simulink model "localMapServer"  (R2024a)
settings: Solver=FixedStepAuto  StartTime=0.0  StopTime=inf  RelTol=1e-3
model workspace (MAT data in the model file):
  SL_ROS_VariableLengthArrays_MaxSizes.CommonInfo.ArrayTruncateAction = 'EmitWarning'
  SL_ROS_VariableLengthArrays_MaxSizes.MsgTypeMap = containers.Map
  SL_ROS_VariableLengthArrays_MaxSizes.MsgTypeMap.serialization.keys = {'std_msgs/Int8MultiArray'}
  SL_ROS_VariableLengthArrays_MaxSizes.MsgTypeMap.serialization.values{1}.PropertyName = 'data'
  SL_ROS_VariableLengthArrays_MaxSizes.MsgTypeMap.serialization.values{1}.DataType = 'int8'
  SL_ROS_VariableLengthArrays_MaxSizes.MsgTypeMap.serialization.values{1}.MaxLength = 1500000
  SL_ROS_VariableLengthArrays_MaxSizes.MsgTypeMap.serialization.uniformity = 0
  SL_ROS_VariableLengthArrays_MaxSizes.MsgTypeMap.serialization.keyType = 'char'
  SL_ROS_VariableLengthArrays_MaxSizes.MsgTypeMap.serialization.valueType = 'any'
undefined symbols (not defined in the file): egogridsize, egomat, egores, gridloc
libraries: roshelperlib x2, ros2lib x2, simulink x1
settings Model: Creator=cstabile  LastModifiedBy=cstabile
settings OptimizationCC: EnhancedBackFolding=on  PassReuseOutputArgsAs=Individual arguments  ZeroExternalMemoryAtStartup=off  ZeroInternalMemoryAtStartup=off  MaxStackSize=64  OptimizeBlockOrder=speed  DifferentSizesBufferReuse=on  OptimizationCustomize=off  EfficientTunableParamExpr=on
settings DebuggingCC: ParameterTunabilityLossMsg=error
settings SFSimCC: MATLABDynamicMemAlloc=off
settings RTWCC: Description=Embedded Coder  SystemTargetFile=ert.tlc  HardwareBoard=Robot Operating System 2 (ROS 2)  TLCOptions="-aInlineSetEventsForThisBaseRateFcn=TLC_FALSE -aSuppressMultiTaskScheduler=TLC_FALSE  -aRateBasedStepFcn=0"  TemplateMakefile=ert_default_tmf  Toolchain=Colcon Tools  TargetLang=C++
settings CodeAppCC: ForceParamTrailComments=on  IgnoreCustomStorageClasses=off  OperatorAnnotations=on  SimulinkDataObjDesc=on  SFDataObjDesc=on  InsertBlockDesc=on
settings ERTTargetCC: CodeInterfacePackaging=C++ class  RootIOFormat=Structure reference

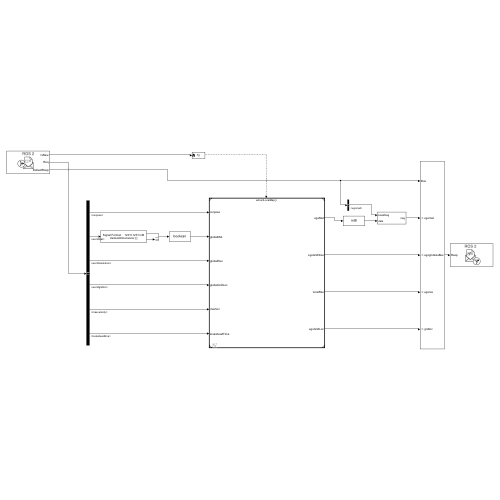
[thumbnail: Simulink's stored preview of the top-level diagram]
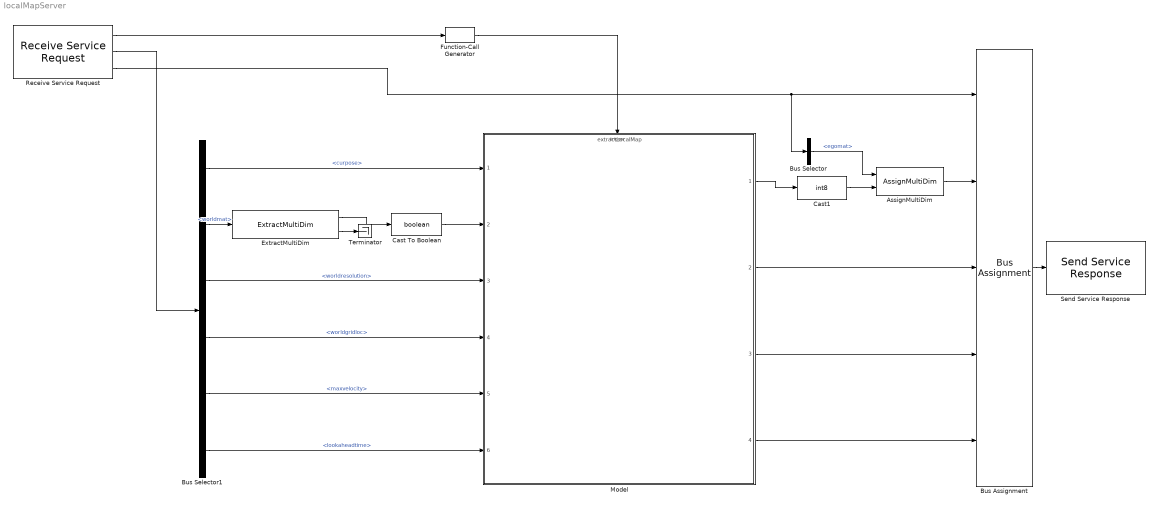
== system localMapServer ==
  AssignMultiDim : roshelperlib/AssignMultiDim  SystemSampleTime=-1  VariantActivationTime=update diagram  AllowFlexibleInterface=on  Latency=0  AutoFrameSizeCalculation=off
  Bus Assignment : BusAssignment  AssignedSignals=egomat,egogridsize,egores,gridloc
  Bus Selector : BusSelector  OutputSignals=egomat
  Bus Selector1 : BusSelector  OutputSignals=curpose,worldmat,worldresolution,worldgridloc,maxvelocity,lookaheadtime
  Cast To Boolean : DataTypeConversion  OutDataTypeStr=boolean  SaturateOnIntegerOverflow=off  RndMeth=Floor
  Cast1 : DataTypeConversion  OutDataTypeStr=int8  SaturateOnIntegerOverflow=off  RndMeth=Floor
  ExtractMultiDim : roshelperlib/ExtractMultiDim  userDataType=int8  dims=[1201 1201]  isVarsize=on  varsizeDims=[]  returnFixedTF=on
  Function-Call Generator : simulink/Ports & Subsystems/Function-Call Generator  sample_time=1  numberOfIterations=1  DisallowWideOutput=off  ShowEnablePort=on
  Model : ModelReference  ModelNameDialog=extractLocalMap.slx  SimulationMode=Normal  ModelReferenceVersion=1.6  TriggerPortName=function  TriggerPortTriggerType=function-call  TriggerPortStatesWhenEnabling=held
  Receive Service Request : ros2lib/Receive Service Request  service=/getlocalmap  serviceType=offroad_msg/ExtractLocalMap  SampleTime=-1  ShowDefaultRespOutput=on  BlockId=ServRec_localMapServer_14  QOSHistory=Keep last  QOSDepth=1  QOSReliability=Reliable  QOSDurability=Volatile  QOSDeadline=Inf  QOSLifespan=Inf  QOSLiveliness=Automatic  QOSLeaseDuration=Inf  QOSAvoidROSNamespaceConventions=off
      settings: LibrarySourceBlock=ros2lib/Receive Request
  Send Service Response : ros2lib/Send Service Response  service=/getlocalmap  serviceType=offroad_msg/ExtractLocalMap  BlockId=ServRec_localMapServer_14
      settings: LibrarySourceBlock=ros2lib/Send Response
  Terminator : Terminator
  wires:
  Function-Call Generator/1 -> Model/Trigger
  Cast1/1 -> AssignMultiDim/2
  Bus Assignment/1 -> Send Service Response/1
  ExtractMultiDim/2 -> Terminator/1
  Receive Service Request/2 -> Bus Selector1/1
  Bus Selector/1 -> AssignMultiDim/1  "<egomat>"
  Receive Service Request/1 -> Function-Call Generator/1
  Bus Selector1/1 -> Model/1  "<curpose>"
  Model/1 -> Cast1/1
  Bus Selector1/2 -> ExtractMultiDim/1  "<worldmat>"
  Receive Service Request/3 -> Bus Assignment/1, Bus Selector/1
  AssignMultiDim/1 -> Bus Assignment/2
  ExtractMultiDim/1 -> Cast To Boolean/1
  Cast To Boolean/1 -> Model/2
  Bus Selector1/3 -> Model/3  "<worldresolution>"
  Bus Selector1/4 -> Model/4  "<worldgridloc>"
  Bus Selector1/5 -> Model/5  "<maxvelocity>"
  Bus Selector1/6 -> Model/6  "<lookaheadtime>"
  Model/2 -> Bus Assignment/3
  Model/3 -> Bus Assignment/4
  Model/4 -> Bus Assignment/5
